simulink model "MovingAvg"  (R2022a)
settings: Solver=FixedStepAuto  StartTime=0.0  StopTime=100  FixedStep=0.001  RelTol=1e-3
undefined symbols (not defined in the file or in its folder): sigbuilder_block
libraries: dspstat3 x1
settings Model: Creator=rupak  LastModifiedBy=rupak
settings ConfigComp: DVTestSuiteOptimization=Auto  DVDetectOutOfBounds=on  DVModelReferenceHarness=on  DVHarnessSource=Signal Editor

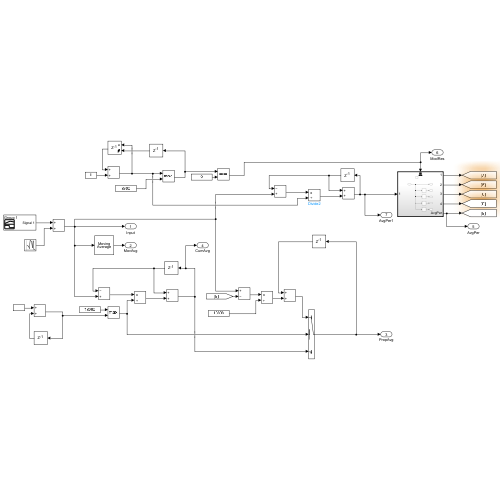
[thumbnail: Simulink's stored preview of the top-level diagram]
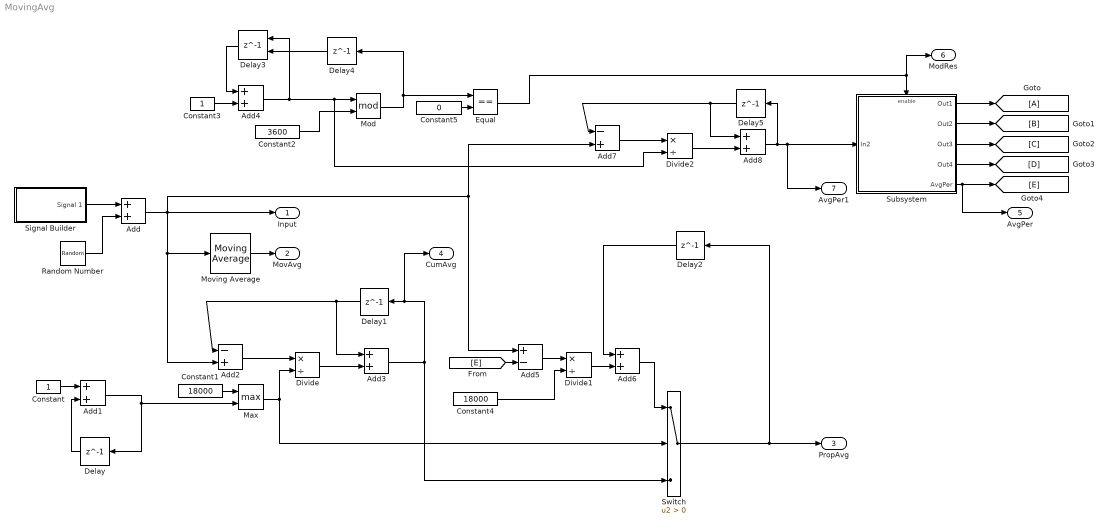
== system MovingAvg ==
  Add{,1,3..4,6,8} (6 alike) : Sum
  Add2 : Sum  Inputs=-+
  Add5 : Sum  Inputs=+-
  Add7 : Sum  Inputs=-+
  Constant : Constant
  Constant1 : Constant  Value=18000
  Constant2 : Constant  Value=3600
  Constant3 : Constant
  Constant4 : Constant  Value=18000
  Constant5 : Constant  Value=0
  Delay{,1..2,4..5} (5 alike) : Delay  DelayLength=1
  Delay3 : Delay  DelayLength=1  ExternalReset=Rising
      settings: InputPortMap=u0,r5
  Divide : Product  Inputs=*/
  Divide1 : Product  Inputs=*/
  Divide2 : Product  Inputs=*/
  Equal : RelationalOperator  Operator===  OutDataTypeStr=boolean  RndMeth=Simplest  InputSameDT=off
  Goto : Goto
  Max : MinMax  Function=max  Inputs=2
  Mod : Math  Operator=mod
  Moving Average : dspstat3/Moving Average  Method=Sliding window  ForgettingFactorPort=off  SpecifyWindowLength=on  WindowLength=18000  ForgettingFactor=0.9  SimulateUsing=Code generation
  Random Number : RandomNumber  Mean=5  SampleTime=0.001
  Signal Builder : Subsystem  Tag=STV Subsys  LoadFcn=sigbuilder_block('load');  StartFcn=sigbuilder_block('start');  StopFcn=sigbuilder_block('stop');  ClipboardFcn=sigbuilder_block('clipboard');  mask(Sigbuilder block){tuvar=[0:10]}
      mask help: Simulink:masks:SigbuilderBlock_MD
      mask init:
      | if ~strcmp(get_param(bdroot(gcbh),'SimulationStatus'),'stopped') tuvar = sigbuilder_block('maskInit'); end
      settings: CopyFcn=sigbuilder_block('copy');  DeleteFcn=sigbuilder_block('delete');  ModelCloseFcn=sigbuilder_block('modelClose');  PreSaveFcn=sigbuilder_block('preSave');  PauseFcn=sigbuilder_block('pause');  ContinueFcn=sigbuilder_block('continue');  NameChangeFcn=sigbuilder_block('namechange');  OpenFcn=sigbuilder_block('open',[6 36 1428 675.75 ]);  CloseFcn=sigbuilder_block('close');
      mask Display: plot(0, 0, 100, 100,[2, 2, 32, 32, 2], [68, 8, 8, 68, 68],[32, 2], [38, 38], [32, 19, 2],[53, 60, 44], [32, 17, 17, 2],[16, 16, 31, 31]);txt = getActiveGroup(gcbh);text(2, 100, txt,'verticalAlignment', 'top');
  Subsystem : Subsystem
  Switch : Switch  Criteria=u2 > Threshold  SaturateOnIntegerOverflow=off  InputSameDT=off
  Input : Outport
  MovAvg : Outport  Port=2
  PropAvg : Outport  Port=3
  CumAvg : Outport  Port=4
  AvgPer : Outport  Port=5
  ModRes : Outport  Port=6
  AvgPer1 : Outport  Port=7
  wires:
  Signal Builder/1(Signal 1) -> Add/1
  Random Number/1 -> Add/2
  Constant/1 -> Add1/1
  Add1/1 -> Delay/1, Max/2
  Delay/1 -> Add1/2
  Moving Average/1 -> MovAvg/1
  Delay1/1 -> Add3/1, Add2/1
  Add2/1 -> Divide/1
  Constant1/1 -> Max/1
  Max/1 -> Switch/2, Divide/2
  Add3/1 -> Switch/3, CumAvg/1, Delay1/1
  Divide/1 -> Add3/2
  Constant2/1 -> Mod/2
  Add4/1 -> Delay3/1, Divide2/2, Mod/1
  Constant3/1 -> Add4/2
  Delay3/1 -> Add4/1
  Subsystem/1(Out1) -> Goto/1
  Subsystem/2(Out2) -> [B]
  Subsystem/3(Out3) -> [C]
  Subsystem/4(Out4) -> [D]
  Subsystem/5(AvgPer) -> AvgPer/1, [E]
  Switch/1 -> PropAvg/1, Delay2/1
  [E] -> Add5/2
  Add5/1 -> Divide1/1
  Constant4/1 -> Divide1/2
  Divide1/1 -> Add6/2
  Delay2/1 -> Add6/1
  Add6/1 -> Switch/1
  Delay4/1 -> Delay3/2
  Equal/1 -> ModRes/1, Subsystem/Enable
  Constant5/1 -> Equal/2
  Mod/1 -> Equal/1, Delay4/1
  Add/1 -> Moving Average/1, Add2/2, Add7/2, Add5/1, Input/1
  Delay5/1 -> Add8/1, Add7/1
  Divide2/1 -> Add8/2
  Add7/1 -> Divide2/1
  Add8/1 -> AvgPer1/1, Subsystem/1(In2), Delay5/1

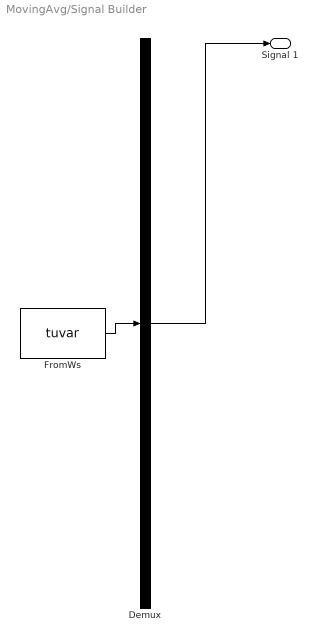
== system MovingAvg/Signal Builder ==
  Demux : Demux  Tag=STV Demux  Outputs=1
      settings: DisplayOption=none
  FromWs : FromWorkspace  Tag=STV FromWs  VariableName=tuvar
      SigBuilderData=|
      | common.afterFinalStr = 'Extrapolate'
      | common.sampleTime = 0
      | dataSet.timeRange = [0 250]
      | dataSet.name = 'Group 1'
      | sbobj.Groups.Name = 'Group 1'
      | sbobj.Groups.Signals.Name = 'Signal 1'
      | sbobj.Groups.Signals.XData = [0 5 5 11 13 16 18.5 21 24.5 31 36.5 40 44 50 57 61 61 65 65 71 75 79 81.5 85.5 87.5 89 89.5 93 98 104 108.4 112.5 121.5 133 145 150.5 154.5 157.5 160 162 165.5 170 176.5 181 182.5 184.5 191 199.5 208 217 231.5 250]
      | sbobj.Groups.Signals.YData = [1 89.6 68.2 83 74 55.8 83.4 73.4 79.8 64.2 90 82.6 66.4 76.4 66 60 47 17.6 30.6 59.6 61.8 47.6 62.4 85.6 77.2 82.2 70 57.4 77.6 35 84.4 56 41 65.6 47 66.6 59.6 72.6 86.4 84.4 55.6 60 33 50.4 73.2 54.8 92 77 59.6 74.6 63 48]
      | sbobj.Groups.TimeRange = [0 250]
  Signal 1 : Outport  Tag=STV Outport
  wires:
  Demux/1 -> Signal 1/1
  FromWs/1 -> Demux/1

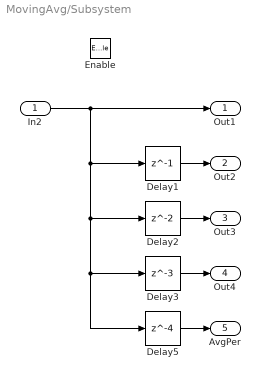
== system MovingAvg/Subsystem ==
  In2 : Inport
  Enable : EnablePort
  Delay1 : Delay  DelayLength=1
  Delay2 : Delay
  Delay3 : Delay  DelayLength=3
  Delay5 : Delay  DelayLength=4
  Out1 : Outport
  Out2 : Outport  Port=2
  Out3 : Outport  Port=3
  Out4 : Outport  Port=4
  AvgPer : Outport  Port=5
  wires:
  Delay1/1 -> Out2/1
  Delay2/1 -> Out3/1
  Delay3/1 -> Out4/1
  Delay5/1 -> AvgPer/1
  In2/1 -> Delay1/1, Delay3/1, Delay5/1, Delay2/1, Out1/1
